simulink model "Lq_Identification_sim_simscape"  (R2026a)
settings: Solver=ode23t  StopTime=t_total(end)
values from neighbouring files (symbols this model uses):
  Beat = 0    [Ld_Identification_m.m]    (also in Lq_Identification_m.m = 1)
  J = 0.00062    [Ld_Identification_m.m]    (also in Lq_Identification_m.m)
  Ld = 2e-3    (= 0.002)    [Ld_Identification_m.m]    (also in Lq_Identification_m.m)
  Lq = 2.5e-3    (= 0.0025)    [Ld_Identification_m.m]    (also in Lq_Identification_m.m)
  np = 14    [Ld_Identification_m.m]    (also in Lq_Identification_m.m)
  Psi = 0.01    [Ld_Identification_m.m]    (also in Lq_Identification_m.m)
  Rs = 8    [Ld_Identification_m.m]    (also in Lq_Identification_m.m)
  Ts = 1/f    (= 6.66666666667e-05)    [Ld_Identification_m.m]    (also in Lq_Identification_m.m)
  Udc = 12    [Ld_Identification_m.m]    (also in Lq_Identification_m.m)
undefined symbols (not defined in the file or in its folder): PermanentMagnetSynchrono_class
libraries: fl_lib x12, nesl_utility x10, ee_lib x4, simulink x3, spsControlledVoltageSourceLib x3, sl_discontinuities x3, eeTransforms x2, elec_conv_HighZElecRef x1
settings Model: Creator=mushen  LastModifiedBy=mushen
settings DebuggingCC: SaveWithParameterizedLinksMsg=none
settings SimscapeCC: SimscapeLogType=none  SimscapeLogDataHistory=5000.0

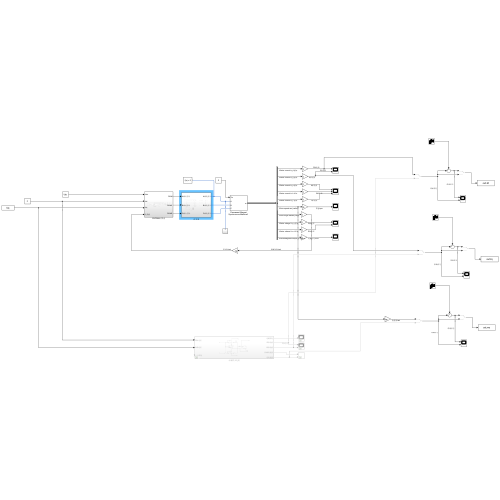
[thumbnail: Simulink's stored preview of the top-level diagram]
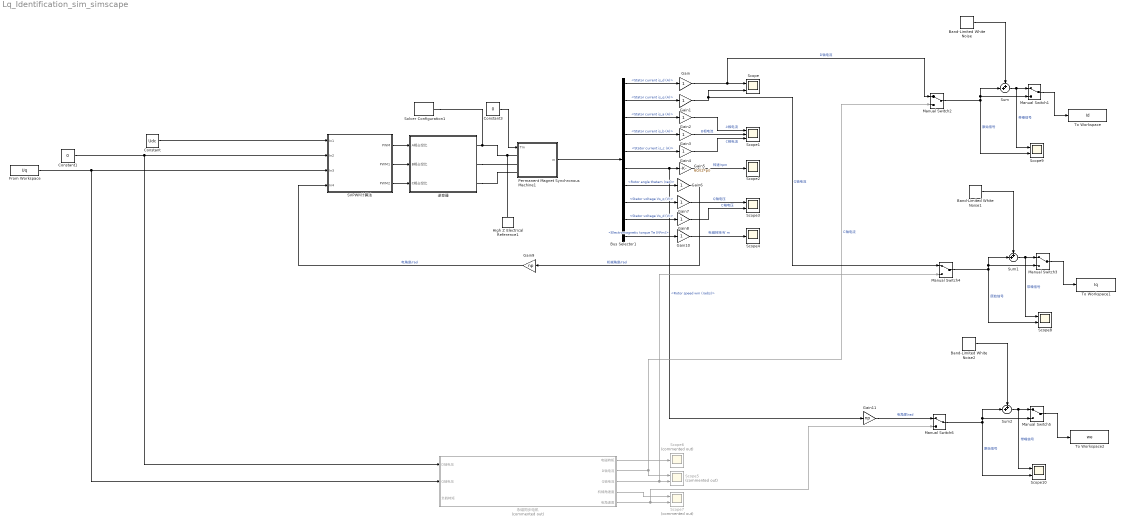
== system Lq_Identification_sim_simscape ==
  Band-Limited White Noise : simulink/Sources/Band-Limited White Noise  Cov=[0.000000005]  Ts=Ts  seed=DC
  Band-Limited White Noise1 : simulink/Sources/Band-Limited White Noise  Cov=[0.000000005]  Ts=Ts  seed=DC
  Band-Limited White Noise2 : simulink/Sources/Band-Limited White Noise  Cov=[0.00001]  Ts=Ts  seed=DC
  Bus Selector1 : BusSelector  OutputSignals=Stator current is_d (A),Stator current is_q (A),Stator current is_a (A),Stator current is_b (A),Stator current is_c (A),Rotor speed wm (rad/s),Rotor angle thetam (rad),Stator voltage Vs_q (V),Stator voltage Vs_d (V),Electromagnetic torque Te (N*m)
  Constant : Constant  Value=Udc
  Constant1 : Constant  Value=0
  Constant3 : Constant  Value=0
  From Workspace : FromWorkspace  VariableName=Uq  SampleTime=Ts
  Gain{,1..4,6..8,10} (9 alike) : Gain
  Gain11 : Gain  Gain=np
  Gain5 : Gain  Gain=60/(2*pi)
  Gain9 : Gain  Gain=np
  High Z Electrical Reference1 : elec_conv_HighZElecRef/High Z Electrical Reference  SystemSampleTime=-1  VariantActivationTime=update diagram  EmptyChoice=off  PassThrough=off  PassThroughVariantControl=(default)  EmptyChoiceVariantControl=(default)  AllowFlexibleInterface=on  Latency=0  AutoFrameSizeCalculation=off
  Manual Switch{1..6} (6 alike) : ManualSwitch
  Permanent Magnet Synchronous Machine1 : Subsystem
      settings: OpenFcn=elec.conv.unmask(gcb);
  SVPWM计算法 : Subsystem
  Scope{,3,8..10} (5 alike) : Scope  NumInputPorts=2
      Scope settings: ActiveDisplayYMinimum=-0.12575  ActiveDisplayYMaximum=0.72199  DataLoggingVariableName=ScopeData2
      Scope10 settings: ActiveDisplayYMinimum=-30.08805  ActiveDisplayYMaximum=265.81147  DataLoggingVariableName=ScopeData12
      Scope3 settings: ActiveDisplayYMinimum=-0.125  ActiveDisplayYMaximum=1.125  DataLoggingVariableName=ScopeData5
      Scope8 settings: ActiveDisplayYMinimum=-0.13328  ActiveDisplayYMaximum=0.74199  DataLoggingVariableName=ScopeData11
      Scope9 settings: ActiveDisplayYMinimum=-0.05353  ActiveDisplayYMaximum=0.11695  DataLoggingVariableName=ScopeData10
  Scope1 : Scope  NumInputPorts=3
      settings: ActiveDisplayYMinimum=-0.72932  ActiveDisplayYMaximum=0.58893  DataLoggingVariableName=ScopeData3
  Scope2 : Scope
      settings: ActiveDisplayYMinimum=-7.33614  ActiveDisplayYMaximum=66.02529  DataLoggingVariableName=ScopeData4
  Scope4 : Scope
      settings: ActiveDisplayYMinimum=-0.14462  ActiveDisplayYMaximum=0.14875  DataLoggingVariableName=ScopeData6
  Scope5 : Scope  Commented=on  NumInputPorts=2
      settings: ActiveDisplayYMinimum=-0.01547  ActiveDisplayYMaximum=0.13925  DataLoggingVariableName=ScopeData7
  Scope6 : Scope  Commented=on
      settings: ActiveDisplayYMinimum=-0.00325  ActiveDisplayYMaximum=0.02924  DataLoggingVariableName=ScopeData8
  Scope7 : Scope  Commented=on  NumInputPorts=2
      settings: ActiveDisplayYMinimum=-11.57862  ActiveDisplayYMaximum=104.20758  DataLoggingVariableName=ScopeData9
  Solver Configuration1 : nesl_utility/Solver Configuration  PhysicalDomain=network_engine_domain  SubClassName=solver  LeftPortType=input  RightPortType=generic  Tones=[]  Harmonics=[]  SimulateNoise=off  Profile=off  UseLocalSampling=off  EnableSwitchedLinearOptims=on  FrequencyDomain=off  UseCCode=off  RelTol=0.001  AbsTol=0.001  MinStep=1e-09  ToWorkspace=off  RevertToSquareIcSolve=off  NumHomotopyIterations=100  PhasorMode=off  PhasorModeNumHarmonics=1  ConsistencySolver=NEWTON_XTOL_AFTER_FTOL  CanonicalOrdering=CANONICAL  OptimizeIntermediates=OPTIMIZED  IndexReductionMethod=DerivativeReplacement  DoDC=off  ResidualTolerance=1e-09  ConsistencyTolSource=GLOBAL  ConsistencyAbsTol=0.001  ConsistencyRelTol=0.001  ConsistencyTolFactor=0.001  UseLocalSolver=off  LocalSolverChoice=NE_BACKWARD_EULER_ADVANCER  ResolveIndetEquations=on  FunctionEvalNumThread=1  LocalSolverSampleTime=0.001  DoFixedCost=off  MaxNonlinIter=3  MaxModeIter=2  ComputeImpulses=off  ImpulseIterations=2  LinearAlgebra=auto  LinearAlgebraNumThread=0  EquationFormulation=NE_TIME_EF  DelaysMemoryBudget=1024  AutomaticFiltering=on  FilteringTimeConstant=0.001  PartitionStorageMethod=AS_NEEDED  PartitionMemoryBudget=1024  PartitionMethod=ROBUST  MultibodyUseLocalSolver=off  MultibodyLocalSolverChoice=ODE1  MultibodyLocalSolverSampleTime=0.001
  Sum : Sum  Inputs=++|
  Sum1 : Sum  Inputs=++|
  Sum2 : Sum  Inputs=++|
  To Workspace : ToWorkspace  VariableName=Id  SaveFormat=Timeseries  SampleTime=Ts
  To Workspace1 : ToWorkspace  VariableName=Iq  SaveFormat=Timeseries  SampleTime=Ts
  To Workspace2 : ToWorkspace  VariableName=we  SaveFormat=Timeseries  SampleTime=Ts
  永磁同步电机 : Subsystem  Commented=on
  逆变器 : Subsystem
  wires:
  Manual Switch1/1 -> To Workspace/1
  Gain8/1 -> Scope3/2  "D轴电压"
  Bus Selector1/10 -> Gain10/1  "<Electromagnetic torque Te (N*m)>"
  Constant1/1 -> 永磁同步电机/1(D轴电压), SVPWM计算法/2(In2)
  Bus Selector1/7 -> Gain6/1  "<Rotor angle thetam (rad)>"
  Bus Selector1/1 -> Gain/1  "<Stator current is_d (A)>"
  Sum/1 -> Scope9/1, Manual Switch1/1  "带噪信号"
  Bus Selector1/2 -> Gain1/1  "<Stator current is_q (A)>"
  Gain5/1 -> Scope2/1  "转速/rpm"
  Bus Selector1/4 -> Gain3/1  "<Stator current is_b (A)>"
  永磁同步电机/4(机械角速度) -> Scope7/1
  Bus Selector1/9 -> Gain8/1  "<Stator voltage Vs_d (V)>"
  Gain4/1 -> Scope1/3  "C相电流"
  SVPWM计算法/2(PWM1) -> 逆变器/2(B相占空比)
  Bus Selector1/6 -> Gain11/1, Gain5/1  "<Rotor speed wm (rad/s)>"
  SVPWM计算法/3(PWM2) -> 逆变器/3(C相占空比)
  Gain3/1 -> Scope1/2  "B相电流"
  永磁同步电机/1(电磁转矩) -> Scope6/1
  Gain6/1 -> Gain9/1  "机械角度/rad"
  永磁同步电机/2(D轴电流) -> Manual Switch2/2, Scope5/1  "D轴电流"
  Gain2/1 -> Scope1/1  "A相电流"
  Permanent Magnet Synchronous Machine1/1(m) -> Bus Selector1/1
  Gain/1 -> Manual Switch2/1, Scope/1  "D轴电流"
  Gain9/1 -> SVPWM计算法/4(In4)  "电角度/rad"
  Bus Selector1/3 -> Gain2/1  "<Stator current is_a (A)>"
  Band-Limited White Noise/1 -> Sum/1
  Constant/1 -> SVPWM计算法/1(In1)
  Bus Selector1/8 -> Gain7/1  "<Stator voltage Vs_q (V)>"
  永磁同步电机/5(电角速度) -> Manual Switch6/2, Scope7/2
  SVPWM计算法/1(PWM) -> 逆变器/1(A相占空比)
  Manual Switch2/1 -> Scope9/2, Manual Switch1/2, Sum/2  "原始信号"
  Gain10/1 -> Scope4/1  "电磁转矩/N`m"
  永磁同步电机/3(Q轴电流) -> Manual Switch4/2, Scope5/2
  Bus Selector1/5 -> Gain4/1  "<Stator current is_c (A)>"
  Gain1/1 -> Manual Switch4/1, Scope/2  "Q轴电流"
  Gain7/1 -> Scope3/1  "Q轴电压"
  Manual Switch4/1 -> Scope8/2, Manual Switch3/2, Sum1/2  "原始信号"
  Band-Limited White Noise1/1 -> Sum1/1
  Manual Switch3/1 -> To Workspace1/1
  Sum1/1 -> Scope8/1, Manual Switch3/1  "带噪信号"
  Manual Switch6/1 -> Scope10/2, Manual Switch5/2, Sum2/2  "原始信号"
  Band-Limited White Noise2/1 -> Sum2/1
  Manual Switch5/1 -> To Workspace2/1
  Sum2/1 -> Scope10/1, Manual Switch5/1  "带噪信号"
  Gain11/1 -> Manual Switch6/1  "电角度/rad"
  From Workspace/1 -> 永磁同步电机/2(Q轴电压), SVPWM计算法/3(In3)
  Constant3/1 -> Permanent Magnet Synchronous Machine1/1(Tm)
  connections:
  逆变器/RConn3 -- Permanent Magnet Synchronous Machine1/LConn3
  逆变器/RConn2 -- Permanent Magnet Synchronous Machine1/LConn2
  逆变器/RConn1 -- Solver Configuration1/RConn1 -- Permanent Magnet Synchronous Machine1/LConn1 -- High Z Electrical Reference1/LConn1

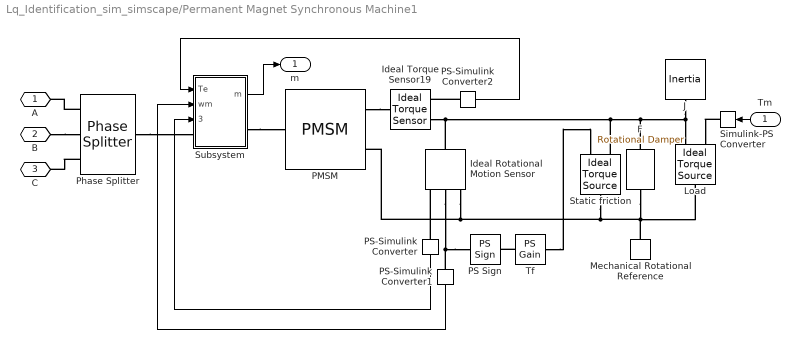
== system Lq_Identification_sim_simscape/Permanent Magnet Synchronous Machine1 ==
  Tm : Inport
  F : fl_lib/Mechanical/Rotational Elements/Rotational Damper  D=0.0003505 N*m/(rad/s)  w_specify=on  w_priority=High  w=0 rad/s  w_nominal_specify=off  w_nominal_value=1  w_nominal_unit=rad/s  t_specify=off  t_priority=None  t=0 N*m  t_nominal_specify=off  t_nominal_value=1  t_nominal_unit=N*m
  Ideal Rotational Motion Sensor : fl_lib/Mechanical/Mechanical Sensors/Ideal Rotational Motion Sensor  reference=foundation.enum.MeasurementReference.difference  acceleration_port=false  velocity_port=true  position_port=true  wrap_angle=simscape.enum.onoff.off  offset=0 deg
  Ideal Torque Sensor19 : fl_lib/Mechanical/Mechanical Sensors/Ideal Torque Sensor
  J : fl_lib/Mechanical/Rotational Elements/Inertia  inertia=J kg*m^2  num_ports=foundation.enum.numPorts2.one  w_specify=on  w_priority=High  w=0 rad/s  w_nominal_specify=off  w_nominal_value=1  w_nominal_unit=rad/s  t_specify=off  t_priority=None  t=0 N*m  t_nominal_specify=off  t_nominal_value=1  t_nominal_unit=N*m
  Load : fl_lib/Mechanical/Mechanical Sources/Ideal Torque Source
  Mechanical Rotational Reference : fl_lib/Mechanical/Rotational Elements/Mechanical Rotational Reference
  PMSM : ee_lib/Electromechanical/Permanent Magnet/PMSM  port_option=ee.enum.threePhasePort.composite  winding_type=ee.enum.statorconnection.wye  machine_param=ee.enum.pmsm.parameterization.constant  nPolePairs=np  pmflux_param=1  pm_flux_linkage=PermanentMagnetSynchrono_class('Torque Tm',[J 0.0003505 np 0],4,'Flux linkage established by magnets (V.s)',Psi,25.3932,0.21,'Aligned with phase A axis (original Park)',[0 0 0 0],'Sinusoidal',120,'3',[0 0 0 0 0 0]).objParamMappingDerived.NewDerivedParam.pm_flux_linkage Wb  torque_constant=0.18 N*m/A  back_emf_constant=0.18 V/(rad/s)  stator_param=1  Ld=Ld H  Lq=Lq H  idVec=[-200, 0, 200] A  iqVec=[-200, 0, 200] A  LdMatrix=0.0002 * ones(3, 3) H  LqMatrix=0.0002 * ones(3, 3) H  PmMatrix=0.1 * ones(3, 3) Wb  ktMatrix=0.18 * ones(3, 3) N*m/A  keMatrix=0.18 * ones(3, 3) V/(rad/s)  L0=1e-09 H  Ls=0.0002 H  Lm=-0.00002 H  Ms=0.00002 H  Rs=Rs Ohm  zero_sequence=0  axes_param=2  loss_param=ee.enum.ironloss.none  losses_oc=[0, 0, 0] W  losses_sc=[0, 0, 0] W  f_losses=60 Hz  Isc_losses=95 A  J=0 kg*m^2  lam=0 N*m/(rad/s)  i_d_specify=on  i_d_priority=High  i_d=PermanentMagnetSynchrono_class('Torque Tm',[J 0.0003505 np 0],4,'Flux linkage established by magnets (V.s)',Psi,25.3932,0.21,'Aligned with phase A axis (original Park)',[0 0 0 0],'Sinusoidal',120,'3',[0 0 0 0 0 0]).objParamMappingDerived.NewDerivedParam.i_d A  i_d_nominal_specify=off  i_d_nominal_value=1  i_d_nominal_unit=A  i_q_specify=on  i_q_priority=High  i_q=PermanentMagnetSynchrono_class('Torque Tm',[J 0.0003505 np 0],4,'Flux linkage established by magnets (V.s)',Psi,25.3932,0.21,'Aligned with phase A axis (original Park)',[0 0 0 0],'Sinusoidal',120,'3',[0 0 0 0 0 0]).objParamMappingDerived.NewDerivedParam.i_q A  i_q_nominal_specify=off  i_q_nominal_value=1  i_q_nominal_unit=A  torque_specify=off  torque_priority=None  torque=0 N*m  torque_nominal_specify=off  torque_nominal_value=1  torque_nominal_unit=N*m  angular_velocity_specify=on  angular_velocity_priority=High  angular_velocity=0 rad/s  angular_velocity_nominal_specify=off  angular_velocity_nominal_value=1  angular_velocity_nominal_unit=rpm  angular_position_specify=on  angular_position_priority=High  angular_position=0 deg  angular_position_nominal_specify=off  angular_position_nominal_value=1  angular_position_nominal_unit=deg  alpha=3.93e-3 1/K  alpha_flux=-0.001 1/K  Tmeas=298.15 K  stator_thermal_mass=100 J/K  rotor_thermal_mass=200 J/K  Rm_percent_rotor=90  Rd_percent_rotor=30  temperatureA_specify=off  temperatureA_priority=High  temperatureA=25 degC  temperatureA_nominal_specify=off  temperatureA_nominal_value=1  temperatureA_nominal_unit=degC  temperatureB_specify=off  temperatureB_priority=High  temperatureB=25 degC  temperatureB_nominal_specify=off  temperatureB_nominal_value=1  temperatureB_nominal_unit=degC  temperatureC_specify=off  temperatureC_priority=High  temperatureC=25 degC  temperatureC_nominal_specify=off  temperatureC_nominal_value=1  temperatureC_nominal_unit=degC  temperatureR_specify=off  temperatureR_priority=High  temperatureR=25 degC  temperatureR_nominal_specify=off  temperatureR_nominal_value=1  temperatureR_nominal_unit=degC
  PS Sign : fl_lib/Physical Signals/Nonlinear Operators/PS Sign
  PS-Simulink Converter : nesl_utility/PS-Simulink Converter  PhysicalDomain=network_engine_domain  SubClassName=ps_output  LeftPortType=input  RightPortType=output  PseudoPeriodic=off  Frequencies=[]  VectorFormat=1-D array  Unit=1  AffineConversion=off
  PS-Simulink Converter1 : nesl_utility/PS-Simulink Converter  PhysicalDomain=network_engine_domain  SubClassName=ps_output  LeftPortType=input  RightPortType=output  PseudoPeriodic=off  Frequencies=[]  VectorFormat=1-D array  Unit=1  AffineConversion=off
  PS-Simulink Converter2 : nesl_utility/PS-Simulink Converter  PhysicalDomain=network_engine_domain  SubClassName=ps_output  LeftPortType=input  RightPortType=output  PseudoPeriodic=off  Frequencies=[]  VectorFormat=1-D array  Unit=1  AffineConversion=off
  Phase Splitter : ee_lib/Connectors & References/Phase Splitter
  Simulink-PS Converter : nesl_utility/Simulink-PS Converter  PhysicalDomain=network_engine_domain  SubClassName=ps_input  LeftPortType=input  RightPortType=output  PseudoPeriodic=off  Frequencies=[]  NoiseDistribution=none  NoiseParameters=[]  Unit=1  AffineConversion=off  FilteringAndDerivatives=provide  SimscapeFilterOrder=1  InputFilterTimeConstant=0.001  UdotUserProvided=0
  Static friction : fl_lib/Mechanical/Mechanical Sources/Ideal Torque Source
  Subsystem : Subsystem
  Tf : fl_lib/Physical Signals/Functions/PS Gain  gain=PermanentMagnetSynchrono_class('Torque Tm',[J 0.0003505 np 0],4,'Flux linkage established by magnets (V.s)',Psi,25.3932,0.21,'Aligned with phase A axis (original Park)',[0 0 0 0],'Sinusoidal',120,'3',[0 0 0 0 0 0]).objParamMappingDerived.NewDerivedParam.Tf
  A : PMIOPort  Side=Left
  B : PMIOPort  Port=2  Side=Left
  C : PMIOPort  Port=3  Side=Left
  m : Outport  VectorParamsAs1DForOutWhenUnconnected=off
  wires:
  PS-Simulink Converter1/1 -> Subsystem/2(wm)
  PS-Simulink Converter/1 -> Subsystem/3(thetam)
  PS-Simulink Converter2/1 -> Subsystem/1(Te)
  Subsystem/1(m) -> m/1
  Tm/1 -> Simulink-PS Converter/1
  connections:
  PS-Simulink Converter2/LConn1 -- Ideal Torque Sensor19/RConn2
  Phase Splitter/LConn1 -- Subsystem/LConn1
  Subsystem/RConn1 -- PMSM/LConn1
  PS-Simulink Converter/LConn1 -- Ideal Rotational Motion Sensor/RConn3
  Tf/RConn1 -- Static friction/RConn1
  PS Sign/LConn1 -- PS-Simulink Converter1/LConn1 -- Ideal Rotational Motion Sensor/RConn2
  Tf/LConn1 -- PS Sign/RConn1
  PMSM/RConn1 -- Ideal Torque Sensor19/LConn1
  Ideal Torque Sensor19/RConn1 -- Static friction/RConn2 -- F/LConn1 -- Load/RConn2 -- J/LConn1 -- Ideal Rotational Motion Sensor/LConn1
  Phase Splitter/RConn3 -- C/RConn1
  Phase Splitter/RConn1 -- A/RConn1
  B/RConn1 -- Phase Splitter/RConn2
  Simulink-PS Converter/RConn1 -- Load/RConn1
  Load/LConn1 -- F/RConn1 -- Static friction/LConn1 -- PMSM/RConn2 -- Ideal Rotational Motion Sensor/RConn1 -- Mechanical Rotational Reference/LConn1

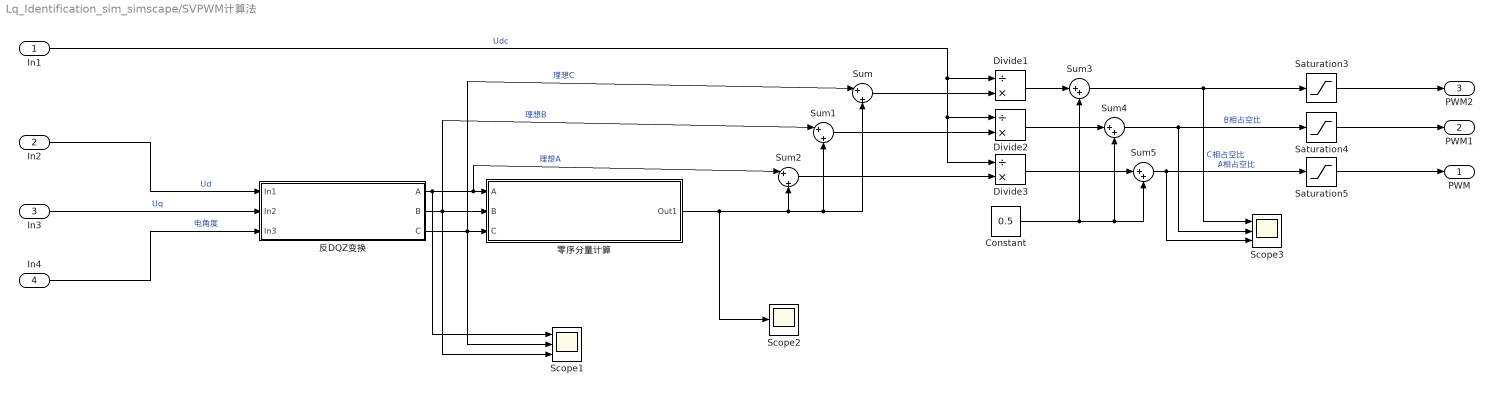
== system Lq_Identification_sim_simscape/SVPWM计算法 ==
  In1 : Inport
  In2 : Inport  Port=2
  In3 : Inport  Port=3
  In4 : Inport  Port=4
  Constant : Constant  Value=0.5
  Divide1 : Product  Inputs=/*
  Divide2 : Product  Inputs=/*
  Divide3 : Product  Inputs=/*
  Saturation3 : Saturate  UpperLimit=1  LowerLimit=0
  Saturation4 : Saturate  UpperLimit=1  LowerLimit=0
  Saturation5 : Saturate  UpperLimit=1  LowerLimit=0
  Scope1 : Scope  NumInputPorts=3
      settings: ActiveDisplayYMinimum=-3.13505  ActiveDisplayYMaximum=3.34432  DataLoggingVariableName=ScopeData2
  Scope2 : Scope
      settings: ActiveDisplayYMinimum=-0.20463  ActiveDisplayYMaximum=-0.00463  DataLoggingVariableName=ScopeData4
  Scope3 : Scope  NumInputPorts=3
      settings: ActiveDisplayYMinimum=0.40979  ActiveDisplayYMaximum=0.59021  DataLoggingVariableName=ScopeData3
  Sum : Sum  Inputs=|+|+
  Sum1 : Sum  Inputs=|+|+
  Sum2 : Sum  Inputs=|+|+
  Sum3 : Sum  Inputs=|++
  Sum4 : Sum  Inputs=|++
  Sum5 : Sum  Inputs=|++
  反DQZ变换 : Subsystem
  零序分量计算 : Subsystem
  PWM : Outport
  PWM1 : Outport  Port=2
  PWM2 : Outport  Port=3
  wires:
  Sum5/1 -> Scope3/3, Saturation5/1  "A相占空比"
  Sum4/1 -> Saturation4/1, Scope3/2  "B相占空比"
  In3/1 -> 反DQZ变换/2(In2)  "Uq"
  In4/1 -> 反DQZ变换/3(In3)  "电角度"
  Sum3/1 -> Scope3/1, Saturation3/1  "C相占空比"
  In2/1 -> 反DQZ变换/1(In1)  "Ud"
  反DQZ变换/1(A) -> Sum2/1, 零序分量计算/1(A), Scope1/1  "理想A"
  反DQZ变换/2(B) -> Sum1/1, Scope1/3, 零序分量计算/2(B)  "理想B"
  反DQZ变换/3(C) -> Sum/1, Scope1/2, 零序分量计算/3(C)  "理想C"
  零序分量计算/1(Out1) -> Sum2/2, Sum/2, Sum1/2, Scope2/1
  Sum2/1 -> Divide3/2
  Sum1/1 -> Divide2/2
  Sum/1 -> Divide1/2
  In1/1 -> Divide3/1, Divide2/1, Divide1/1  "Udc"
  Divide1/1 -> Sum3/1
  Divide3/1 -> Sum5/1
  Divide2/1 -> Sum4/1
  Constant/1 -> Sum3/2, Sum4/2, Sum5/2
  Saturation4/1 -> PWM1/1
  Saturation3/1 -> PWM2/1
  Saturation5/1 -> PWM/1

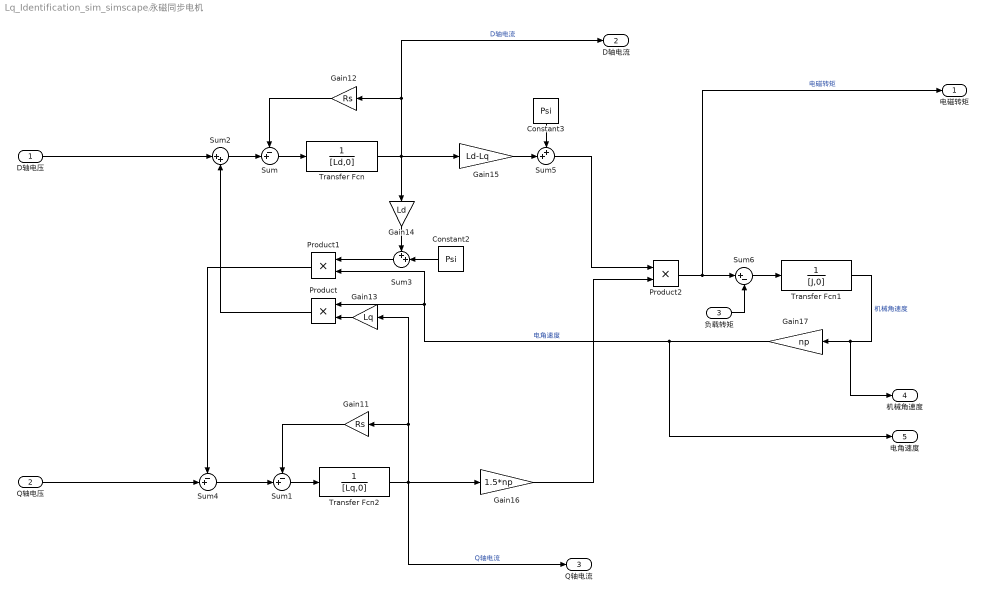
== system Lq_Identification_sim_simscape/永磁同步电机 ==
  D轴电压 : Inport
  Q轴电压 : Inport  Port=2
  负载转矩 : Inport  Port=3
  Constant2 : Constant  Value=Psi
  Constant3 : Constant  Value=Psi
  Gain11 : Gain  Gain=Rs
  Gain12 : Gain  Gain=Rs
  Gain13 : Gain  Gain=Lq
  Gain14 : Gain  Gain=Ld
  Gain15 : Gain  Gain=Ld-Lq
  Gain16 : Gain  Gain=1.5*np
  Gain17 : Gain  Gain=np
  Product : Product
  Product1 : Product
  Product2 : Product
  Sum : Sum  Inputs=-+|
  Sum1 : Sum  Inputs=-+|
  Sum2 : Sum  Inputs=|++
  Sum3 : Sum  Inputs=++|
  Sum4 : Sum  Inputs=-+|
  Sum5 : Sum  Inputs=++|
  Sum6 : Sum  Inputs=|+-
  Transfer Fcn : TransferFcn  Denominator=[Ld,0]
  Transfer Fcn1 : TransferFcn  Denominator=[J,0]
  Transfer Fcn2 : TransferFcn  Denominator=[Lq,0]
  电磁转矩 : Outport
  D轴电流 : Outport  Port=2
  Q轴电流 : Outport  Port=3
  机械角速度 : Outport  Port=4
  电角速度 : Outport  Port=5
  wires:
  Constant2/1 -> Sum3/2
  Gain16/1 -> Product2/2
  Product/1 -> Sum2/2
  Gain17/1 -> 电角速度/1, Product1/2, Product/1  "电角速度"
  Gain12/1 -> Sum/1
  Gain15/1 -> Sum5/2
  Transfer Fcn/1 -> D轴电流/1, Gain12/1, Gain15/1, Gain14/1  "D轴电流"
  Product1/1 -> Sum4/1
  Transfer Fcn2/1 -> Q轴电流/1, Gain16/1, Gain13/1, Gain11/1  "Q轴电流"
  Q轴电压/1 -> Sum4/2
  Constant3/1 -> Sum5/1
  Sum4/1 -> Sum1/2
  Sum3/1 -> Product1/1
  Sum6/1 -> Transfer Fcn1/1
  Sum2/1 -> Sum/2
  Sum1/1 -> Transfer Fcn2/1
  Product2/1 -> 电磁转矩/1, Sum6/1  "电磁转矩"
  D轴电压/1 -> Sum2/1
  Gain14/1 -> Sum3/1
  Sum5/1 -> Product2/1
  Sum/1 -> Transfer Fcn/1
  Gain13/1 -> Product/2
  Transfer Fcn1/1 -> 机械角速度/1, Gain17/1  "机械角速度"
  Gain11/1 -> Sum1/1
  负载转矩/1 -> Sum6/2

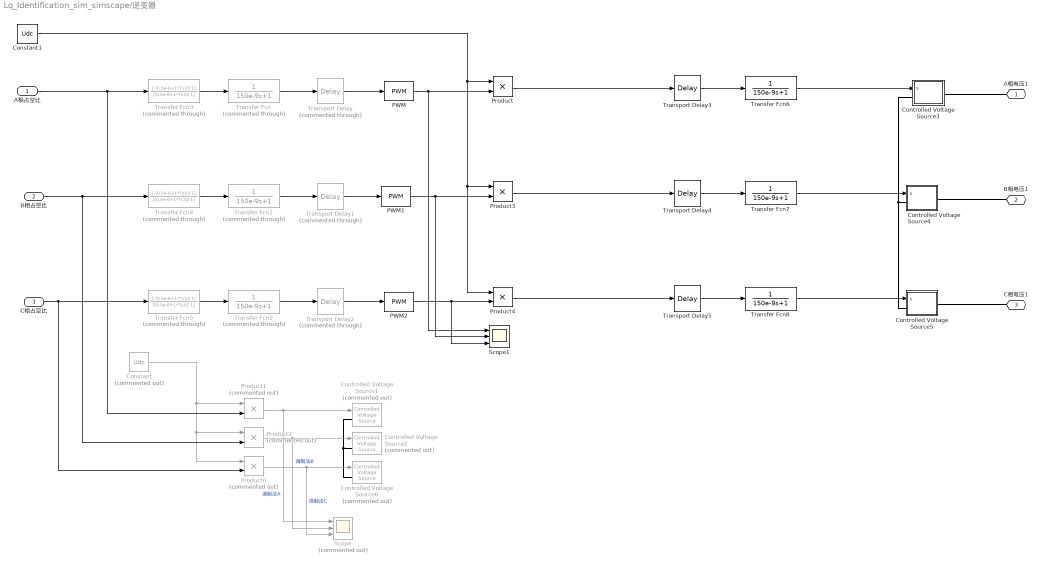
== system Lq_Identification_sim_simscape/逆变器 ==
  A相占空比 : Inport
  B相占空比 : Inport  Port=2
  C相占空比 : Inport  Port=3
  Constant : Constant  Commented=on  Value=Udc
  Constant1 : Constant  Value=Udc
  Controlled Voltage Source1 : spsControlledVoltageSourceLib/Controlled Voltage Source  Commented=on  Initialize=on  Source_Type=DC  Amplitude=0  Phase=0  Frequency=0  Measurements=None
  Controlled Voltage Source2 : spsControlledVoltageSourceLib/Controlled Voltage Source  Commented=on  Initialize=on  Source_Type=DC  Amplitude=0  Phase=0  Frequency=0  Measurements=None
  Controlled Voltage Source3 : Subsystem
  Controlled Voltage Source4 : Subsystem
      settings: OpenFcn=elec.conv.unmask(gcb);
  Controlled Voltage Source5 : Subsystem
      settings: OpenFcn=elec.conv.unmask(gcb);
  Controlled Voltage Source6 : spsControlledVoltageSourceLib/Controlled Voltage Source  Commented=on  Initialize=on  Source_Type=DC  Amplitude=0  Phase=0  Frequency=0  Measurements=None
  PWM : sl_discontinuities/PWM  DisableCoverage=on  Period=Ts  InitialDelay=Beat*Ts  DisallowZeroDutyCycle=off  RunAtFixedTimeIntervals=off  SampleTime=Ts
  PWM1 : sl_discontinuities/PWM  DisableCoverage=on  Period=Ts  InitialDelay=Beat*Ts  DisallowZeroDutyCycle=off  RunAtFixedTimeIntervals=off  SampleTime=Ts
  PWM2 : sl_discontinuities/PWM  DisableCoverage=on  Period=Ts  InitialDelay=Beat*Ts  DisallowZeroDutyCycle=off  RunAtFixedTimeIntervals=off  SampleTime=Ts
  Product : Product
  Product1 : Product  Commented=on
  Product2 : Product  Commented=on
  Product3 : Product
  Product4 : Product
  Product6 : Product  Commented=on
  Scope : Scope  Commented=on  NumInputPorts=3
      settings: ActiveDisplayYMinimum=5.0625  ActiveDisplayYMaximum=6.9375  DataLoggingVariableName=ScopeData4
  Scope1 : Scope  NumInputPorts=3
      settings: ActiveDisplayYMinimum=-0.125  ActiveDisplayYMaximum=1.125
  Transfer Fcn : TransferFcn  Commented=through  Denominator=[150e-9 1]
  Transfer Fcn1 : TransferFcn  Commented=through  Denominator=[150e-9 1]
  Transfer Fcn2 : TransferFcn  Commented=through  Denominator=[150e-9 1]
  Transfer Fcn3 : TransferFcn  Commented=through  Numerator=[-(0.5e-6+1*Ts)/2 1]  Denominator=[(0.5e-6+1*Ts)/2 1]
  Transfer Fcn4 : TransferFcn  Commented=through  Numerator=[-(0.5e-6+1*Ts)/2 1]  Denominator=[(0.5e-6+1*Ts)/2 1]
  Transfer Fcn5 : TransferFcn  Commented=through  Numerator=[-(0.5e-6+1*Ts)/2 1]  Denominator=[(0.5e-6+1*Ts)/2 1]
  Transfer Fcn6 : TransferFcn  Denominator=[150e-9 1]
  Transfer Fcn7 : TransferFcn  Denominator=[150e-9 1]
  Transfer Fcn8 : TransferFcn  Denominator=[150e-9 1]
  Transport Delay : TransportDelay  Commented=through  DelayTime=0.5e-6+1*Ts  TransDelayFeedthrough=on  PadeOrder=1
  Transport Delay1 : TransportDelay  Commented=through  DelayTime=0.5e-6+1*Ts  TransDelayFeedthrough=on  PadeOrder=1
  Transport Delay2 : TransportDelay  Commented=through  DelayTime=0.5e-6+1*Ts  TransDelayFeedthrough=on  PadeOrder=1
  Transport Delay3 : TransportDelay  DelayTime=0.5e-6  TransDelayFeedthrough=on  PadeOrder=1
  Transport Delay4 : TransportDelay  DelayTime=0.5e-6  TransDelayFeedthrough=on  PadeOrder=1
  Transport Delay5 : TransportDelay  DelayTime=0.5e-6  TransDelayFeedthrough=on  PadeOrder=1
  A相电压1 : PMIOPort  Side=Right
  B相电压1 : PMIOPort  Port=2  Side=Right
  C相电压1 : PMIOPort  Port=3  Side=Right
  wires:
  Transfer Fcn/1 -> Transport Delay/1
  Transfer Fcn1/1 -> Transport Delay1/1
  Transport Delay1/1 -> PWM1/1
  Transfer Fcn2/1 -> Transport Delay2/1
  Transport Delay2/1 -> PWM2/1
  Transfer Fcn3/1 -> Transfer Fcn/1
  Transfer Fcn4/1 -> Transfer Fcn1/1
  Transfer Fcn5/1 -> Transfer Fcn2/1
  Constant/1 -> Product1/1, Product6/1, Product2/1
  Product1/1 -> Scope/1, Controlled Voltage Source1/1  "调制法A"
  A相占空比/1 -> Product1/2, Transfer Fcn3/1
  C相占空比/1 -> Product6/2, Transfer Fcn5/1
  Product6/1 -> Scope/3, Controlled Voltage Source6/1  "调制法C"
  Product2/1 -> Scope/2, Controlled Voltage Source2/1  "调制法B"
  B相占空比/1 -> Product2/2, Transfer Fcn4/1
  PWM/1 -> Scope1/1, Product/2
  PWM1/1 -> Scope1/2, Product3/2
  PWM2/1 -> Product4/2, Scope1/3
  Transport Delay/1 -> PWM/1
  Constant1/1 -> Product4/1, Product3/1, Product/1
  Transport Delay3/1 -> Transfer Fcn6/1
  Product/1 -> Transport Delay3/1
  Transport Delay4/1 -> Transfer Fcn7/1
  Transport Delay5/1 -> Transfer Fcn8/1
  Product4/1 -> Transport Delay5/1
  Product3/1 -> Transport Delay4/1
  Transfer Fcn6/1 -> Controlled Voltage Source3/1(s)
  Transfer Fcn7/1 -> Controlled Voltage Source4/1(s)
  Transfer Fcn8/1 -> Controlled Voltage Source5/1(s)
  connections:
  Controlled Voltage Source2/LConn1 -- Controlled Voltage Source6/LConn1 -- Controlled Voltage Source1/LConn1
  B相电压1/RConn1 -- Controlled Voltage Source4/RConn1
  A相电压1/RConn1 -- Controlled Voltage Source3/RConn1
  Controlled Voltage Source5/RConn1 -- C相电压1/RConn1
  Controlled Voltage Source3/LConn1 -- Controlled Voltage Source4/LConn1 -- Controlled Voltage Source5/LConn1

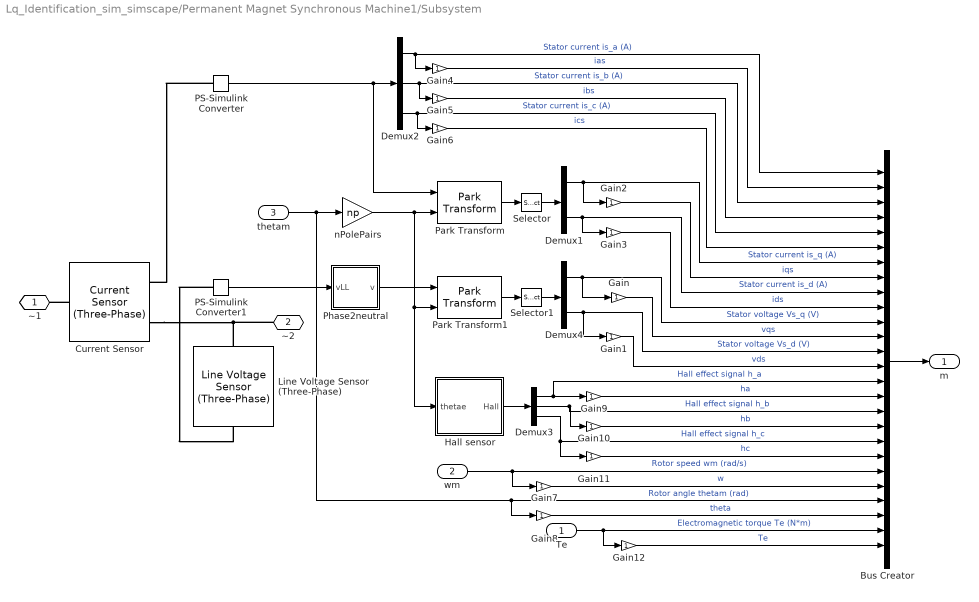
== system Lq_Identification_sim_simscape/Permanent Magnet Synchronous Machine1/Subsystem ==
  Te : Inport
  wm : Inport  Port=2
  thetam : Inport  Port=3
  Bus Creator : BusCreator  Inputs=26
  Current Sensor : ee_lib/Sensors & Transducers/Current Sensor (Three-Phase)  port_option=ee.enum.threePhasePort.composite
  Demux1 : Demux  Outputs=2
  Demux2 : Demux  Outputs=3
  Demux3 : Demux  Outputs=3
  Demux4 : Demux  Outputs=2
  Gain{,1..12} (13 alike) : Gain
  Hall sensor : Subsystem
  Line Voltage Sensor (Three-Phase) : ee_lib/Sensors & Transducers/Line Voltage Sensor (Three-Phase)  port_option=ee.enum.threePhasePort.composite
  PS-Simulink Converter : nesl_utility/PS-Simulink Converter  PhysicalDomain=network_engine_domain  SubClassName=ps_output  LeftPortType=input  RightPortType=output  PseudoPeriodic=off  Frequencies=[]  VectorFormat=1-D array  Unit=1  AffineConversion=off
  PS-Simulink Converter1 : nesl_utility/PS-Simulink Converter  PhysicalDomain=network_engine_domain  SubClassName=ps_output  LeftPortType=input  RightPortType=output  PseudoPeriodic=off  Frequencies=[]  VectorFormat=1-D array  Unit=1  AffineConversion=off
  Park Transform : eeTransforms/Park Transform  AxisAlignment=D-axis  PowerInvariant=off
  Park Transform1 : eeTransforms/Park Transform  AxisAlignment=D-axis  PowerInvariant=off
  Phase2neutral : Subsystem
  Selector : Selector  InputPortWidth=3  IndexOptions=Index vector (dialog)  Indices=[2 1]  OutputSizes=1
  Selector1 : Selector  InputPortWidth=3  IndexOptions=Index vector (dialog)  Indices=[2 1]  OutputSizes=1
  nPolePairs : Gain  Gain=np
  ~1 : PMIOPort  Side=Left
  ~2 : PMIOPort  Port=2  Side=Right
  m : Outport  VectorParamsAs1DForOutWhenUnconnected=off
  wires:
  Phase2neutral/1(v) -> Park Transform1/1
  Gain8/1 -> Bus Creator/24  "theta"
  Gain7/1 -> Bus Creator/22  "w"
  Selector1/1 -> Demux4/1
  Selector/1 -> Demux1/1
  Gain11/1 -> Bus Creator/20  "hc"
  Gain10/1 -> Bus Creator/18  "hb"
  Gain9/1 -> Bus Creator/16  "ha"
  Gain1/1 -> Bus Creator/14  "vds"
  Gain/1 -> Bus Creator/12  "vqs"
  Gain3/1 -> Bus Creator/10  "ids"
  Gain2/1 -> Bus Creator/8  "iqs"
  Hall sensor/1(Hall) -> Demux3/1
  PS-Simulink Converter1/1 -> Phase2neutral/1(vLL)
  Gain6/1 -> Bus Creator/6  "ics"
  Gain5/1 -> Bus Creator/4  "ibs"
  Gain4/1 -> Bus Creator/2  "ias"
  PS-Simulink Converter/1 -> Demux2/1, Park Transform/1
  Te/1 -> Bus Creator/25, Gain12/1  "Electromagnetic torque Te (N*m)"
  Gain12/1 -> Bus Creator/26  "Te"
  Demux3/3 -> Bus Creator/19, Gain11/1  "Hall effect signal h_c"
  Demux3/2 -> Gain10/1, Bus Creator/17  "Hall effect signal h_b"
  Demux3/1 -> Gain9/1, Bus Creator/15  "Hall effect signal h_a"
  thetam/1 -> nPolePairs/1, Gain8/1, Bus Creator/23  "Rotor angle thetam (rad)"
  Bus Creator/1 -> m/1
  Demux2/3 -> Bus Creator/5, Gain6/1  "Stator current is_c (A)"
  Demux2/2 -> Gain5/1, Bus Creator/3  "Stator current is_b (A)"
  Demux2/1 -> Gain4/1, Bus Creator/1  "Stator current is_a (A)"
  Demux1/2 -> Gain3/1, Bus Creator/9  "Stator current is_d (A)"
  Park Transform/1 -> Selector/1
  Demux1/1 -> Gain2/1, Bus Creator/7  "Stator current is_q (A)"
  Demux4/2 -> Gain1/1, Bus Creator/13  "Stator voltage Vs_d (V)"
  Demux4/1 -> Gain/1, Bus Creator/11  "Stator voltage Vs_q (V)"
  Park Transform1/1 -> Selector1/1
  nPolePairs/1 -> Hall sensor/1(thetae), Park Transform1/2, Park Transform/2
  wm/1 -> Bus Creator/21, Gain7/1  "Rotor speed wm (rad/s)"
  connections:
  PS-Simulink Converter1/LConn1 -- Line Voltage Sensor (Three-Phase)/RConn1
  PS-Simulink Converter/LConn1 -- Current Sensor/RConn1
  ~2/RConn1 -- Line Voltage Sensor (Three-Phase)/LConn1 -- Current Sensor/RConn2
  Current Sensor/LConn1 -- ~1/RConn1

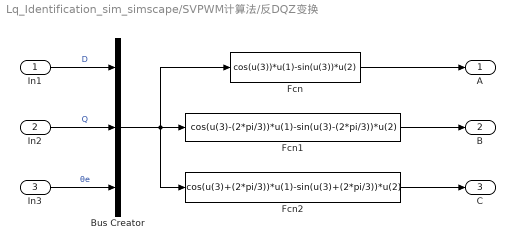
== system Lq_Identification_sim_simscape/SVPWM计算法/反DQZ变换 ==
  In1 : Inport
  In2 : Inport  Port=2
  In3 : Inport  Port=3
  Bus Creator : BusCreator  Inputs=3
  Fcn : Fcn  Expr=cos(u(3))*u(1)-sin(u(3))*u(2)
  Fcn1 : Fcn  Expr=cos(u(3)-(2*pi/3))*u(1)-sin(u(3)-(2*pi/3))*u(2)
  Fcn2 : Fcn  Expr=cos(u(3)+(2*pi/3))*u(1)-sin(u(3)+(2*pi/3))*u(2)
  A : Outport
  B : Outport  Port=2
  C : Outport  Port=3
  wires:
  In3/1 -> Bus Creator/3  "θe"
  In2/1 -> Bus Creator/2  "Q"
  In1/1 -> Bus Creator/1  "D"
  Bus Creator/1 -> Fcn/1, Fcn1/1, Fcn2/1
  Fcn/1 -> A/1
  Fcn1/1 -> B/1
  Fcn2/1 -> C/1

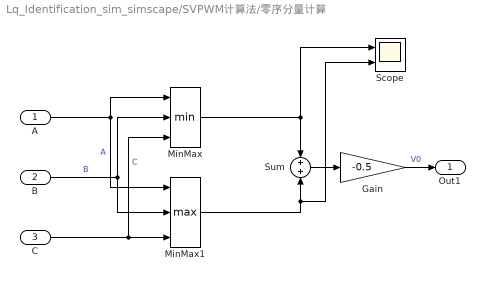
== system Lq_Identification_sim_simscape/SVPWM计算法/零序分量计算 ==
  A : Inport
  B : Inport  Port=2
  C : Inport  Port=3
  Gain : Gain  Gain=-0.5
  MinMax : MinMax  Inputs=3
  MinMax1 : MinMax  Function=max  Inputs=3
  Scope : Scope  NumInputPorts=2
      settings: ActiveDisplayYMinimum=-3.75  ActiveDisplayYMaximum=3.75  DataLoggingVariableName=ScopeData3
  Sum : Sum
  Out1 : Outport
  wires:
  A/1 -> MinMax/1, MinMax1/1  "A"
  B/1 -> MinMax1/2, MinMax/2  "B"
  C/1 -> MinMax/3, MinMax1/3  "C"
  MinMax/1 -> Sum/1, Scope/1
  MinMax1/1 -> Scope/2, Sum/2
  Sum/1 -> Gain/1
  Gain/1 -> Out1/1  "V0"

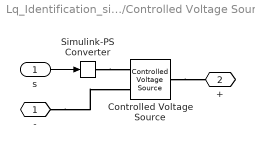
== system Lq_Identification_sim_simscape/逆变器/Controlled Voltage Source3 ==
  s : Inport
  Controlled Voltage Source : fl_lib/Electrical/Electrical Sources/Controlled Voltage Source
  Simulink-PS Converter : nesl_utility/Simulink-PS Converter  PhysicalDomain=network_engine_domain  SubClassName=ps_input  LeftPortType=input  RightPortType=output  PseudoPeriodic=off  Frequencies=[]  NoiseDistribution=none  NoiseParameters=[]  Unit=1  AffineConversion=off  FilteringAndDerivatives=provide  SimscapeFilterOrder=1  InputFilterTimeConstant=0.001  UdotUserProvided=0
  - : PMIOPort  Side=Left
  + : PMIOPort  Port=2  Side=Right
  wires:
  s/1 -> Simulink-PS Converter/1
  connections:
  -/RConn1 -- Controlled Voltage Source/RConn2
  Simulink-PS Converter/RConn1 -- Controlled Voltage Source/RConn1
  Controlled Voltage Source/LConn1 -- +/RConn1

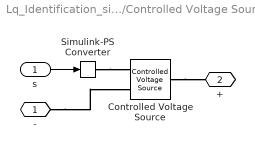
== system Lq_Identification_sim_simscape/逆变器/Controlled Voltage Source4 ==
  s : Inport
  Controlled Voltage Source : fl_lib/Electrical/Electrical Sources/Controlled Voltage Source
  Simulink-PS Converter : nesl_utility/Simulink-PS Converter  PhysicalDomain=network_engine_domain  SubClassName=ps_input  LeftPortType=input  RightPortType=output  PseudoPeriodic=off  Frequencies=[]  NoiseDistribution=none  NoiseParameters=[]  Unit=1  AffineConversion=off  FilteringAndDerivatives=provide  SimscapeFilterOrder=1  InputFilterTimeConstant=0.001  UdotUserProvided=0
  - : PMIOPort  Side=Left
  + : PMIOPort  Port=2  Side=Right
  wires:
  s/1 -> Simulink-PS Converter/1
  connections:
  -/RConn1 -- Controlled Voltage Source/RConn2
  Simulink-PS Converter/RConn1 -- Controlled Voltage Source/RConn1
  Controlled Voltage Source/LConn1 -- +/RConn1

== system Lq_Identification_sim_simscape/逆变器/Controlled Voltage Source5 ==
  s : Inport
  Controlled Voltage Source : fl_lib/Electrical/Electrical Sources/Controlled Voltage Source
  Simulink-PS Converter : nesl_utility/Simulink-PS Converter  PhysicalDomain=network_engine_domain  SubClassName=ps_input  LeftPortType=input  RightPortType=output  PseudoPeriodic=off  Frequencies=[]  NoiseDistribution=none  NoiseParameters=[]  Unit=1  AffineConversion=off  FilteringAndDerivatives=provide  SimscapeFilterOrder=1  InputFilterTimeConstant=0.001  UdotUserProvided=0
  - : PMIOPort  Side=Left
  + : PMIOPort  Port=2  Side=Right
  wires:
  s/1 -> Simulink-PS Converter/1
  connections:
  -/RConn1 -- Controlled Voltage Source/RConn2
  Simulink-PS Converter/RConn1 -- Controlled Voltage Source/RConn1
  Controlled Voltage Source/LConn1 -- +/RConn1

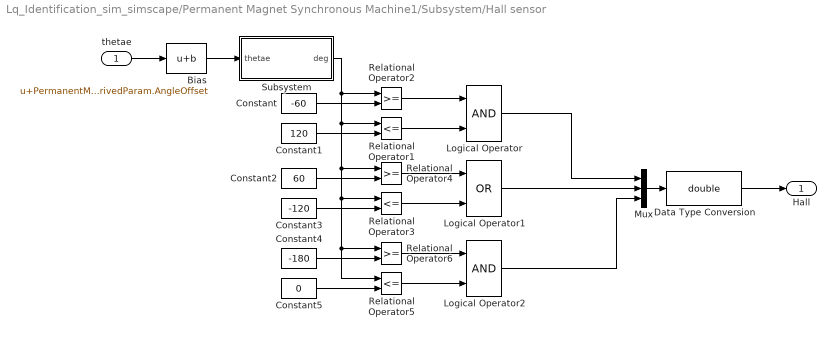
== system Lq_Identification_sim_simscape/Permanent Magnet Synchronous Machine1/Subsystem/Hall sensor ==
  thetae : Inport
  Bias : Bias  Bias=PermanentMagnetSynchrono_class('Torque Tm',[J 0.0003505 np 0],4,'Flux linkage established by magnets (V.s)',Psi,25.3932,0.21,'Aligned with phase A axis (original Park)',[0 0 0 0],'Sinusoidal',120,'3',[0 0 0 0 0 0]).objParamMappingDerived.NewDerivedParam.AngleOffset  SaturateOnIntegerOverflow=off
  Constant : Constant  Value=-60
  Constant1 : Constant  Value=120
  Constant2 : Constant  Value=60
  Constant3 : Constant  Value=-120
  Constant4 : Constant  Value=-180
  Constant5 : Constant  Value=0
  Data Type Conversion : DataTypeConversion  OutDataTypeStr=double  SaturateOnIntegerOverflow=off  RndMeth=Floor
  Logical Operator : Logic  AllPortsSameDT=off  OutDataTypeStr=boolean
  Logical Operator1 : Logic  Operator=OR  AllPortsSameDT=off  OutDataTypeStr=boolean
  Logical Operator2 : Logic  AllPortsSameDT=off  OutDataTypeStr=boolean
  Mux : Mux  Inputs=3
  Relational Operator1 : RelationalOperator  Operator=<=
  Relational Operator2 : RelationalOperator
  Relational Operator3 : RelationalOperator  Operator=<=
  Relational Operator4 : RelationalOperator
  Relational Operator5 : RelationalOperator  Operator=<=
  Relational Operator6 : RelationalOperator
  Subsystem : Subsystem
  Hall : Outport  VectorParamsAs1DForOutWhenUnconnected=off
  wires:
  Bias/1 -> Subsystem/1(thetae)
  Data Type Conversion/1 -> Hall/1
  thetae/1 -> Bias/1
  Constant2/1 -> Relational Operator4/2
  Constant1/1 -> Relational Operator1/2
  Relational Operator4/1 -> Logical Operator1/1
  Constant/1 -> Relational Operator2/2
  Subsystem/1(deg) -> Relational Operator2/1, Relational Operator1/1, Relational Operator6/1, Relational Operator5/1, Relational Operator3/1, Relational Operator4/1
  Relational Operator1/1 -> Logical Operator/2
  Relational Operator2/1 -> Logical Operator/1
  Mux/1 -> Data Type Conversion/1
  Relational Operator3/1 -> Logical Operator1/2
  Constant5/1 -> Relational Operator5/2
  Constant4/1 -> Relational Operator6/2
  Relational Operator6/1 -> Logical Operator2/1
  Relational Operator5/1 -> Logical Operator2/2
  Logical Operator/1 -> Mux/1
  Logical Operator1/1 -> Mux/2
  Logical Operator2/1 -> Mux/3
  Constant3/1 -> Relational Operator3/2

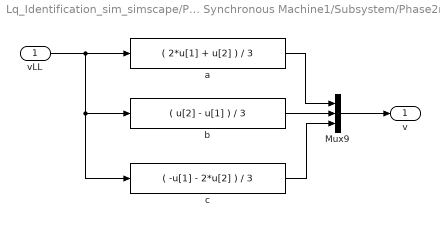
== system Lq_Identification_sim_simscape/Permanent Magnet Synchronous Machine1/Subsystem/Phase2neutral ==
  vLL : Inport
  Mux9 : Mux  Inputs=3
  a : Fcn  Expr=( 2*u[1] + u[2] ) / 3
  b : Fcn  Expr=( u[2] - u[1] ) / 3
  c : Fcn  Expr=( -u[1] - 2*u[2] ) / 3
  v : Outport
  wires:
  b/1 -> Mux9/2
  vLL/1 -> b/1, c/1, a/1
  c/1 -> Mux9/3
  a/1 -> Mux9/1
  Mux9/1 -> v/1

== system Lq_Identification_sim_simscape/Permanent Magnet Synchronous Machine1/Subsystem/Hall sensor/Subsystem ==
  thetae : Inport
  Trigonometric Function : Trigonometry  Operator=sincos
  Trigonometric Function2 : Trigonometry  Operator=atan2
  rad->deg : Gain  Gain=180/pi  SaturateOnIntegerOverflow=on  OutDataTypeStr=Inherit: Same as input  ParamDataTypeStr=Inherit: Same as input
  deg : Outport  VectorParamsAs1DForOutWhenUnconnected=off
  wires:
  thetae/1 -> Trigonometric Function/1
  Trigonometric Function/2 -> Trigonometric Function2/2
  rad->deg/1 -> deg/1
  Trigonometric Function/1 -> Trigonometric Function2/1
  Trigonometric Function2/1 -> rad->deg/1
